simulink model "sergio_arm"  (Simulink 8.5)
settings: Solver=ode45  StartTime=0.0  StopTime=10.0  RelTol=1e-3
undefined symbols (not defined in the file): CPT_w1, GR_w1
libraries: SOEM_EtherCAT_Lib x3
settings Model: Creator=baetenmjj  LastModifiedBy=baetenmjj
settings DataIOCC: SignalLoggingSaveFormat=Dataset
settings OptimizationCC: ExpressionDepthLimit=128
settings DebuggingCC: UnderspecifiedInitializationDetection=Simplified  MergeDetectMultiDrivingBlocksExec=error  FcnCallInpInsideContextMsg=EnableAllAsError  StateNameClashWarn=none
settings GRTTargetCC: CombineOutputUpdateFcns=on  GRTInterface=off

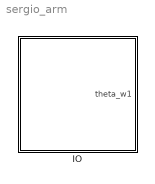
== system sergio_arm ==
  IO : Subsystem

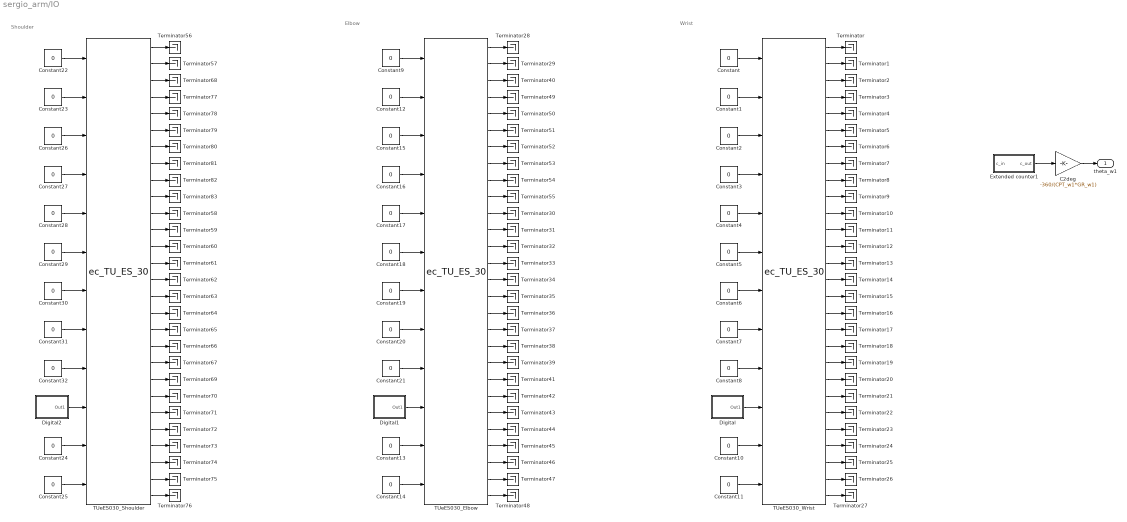
== system sergio_arm/IO ==
  note: Shoulder
  note: Wrist
  note: Elbow
  C2deg : Gain  Gain=-360/(CPT_w1*GR_w1)
  Constant{,1..32} (33 alike) : Constant  Value=0
  Digital : Subsystem
  Digital1 : Subsystem
  Digital2 : Subsystem
  Extended counter1 : Subsystem
  TUeES030_Elbow : SOEM_EtherCAT_Lib/ec_TU_ES_30  link_id=2  slave_num=3  resistance=[1.511, 1.53+0.45*2, 1.53+0.45*2]  kv=[0.0259, 0.0208, 0.0208]  pgain=[4.00, 4.00, 4.00]  igain=[50.00, 50.00, 50.00]  ilimit=[1.0, 1.0, 1.0]  encdir=[1, 1, 1]  encres=[2000, 500, 500]  czero=[17330, 8633, 8522]
  TUeES030_Shoulder : SOEM_EtherCAT_Lib/ec_TU_ES_30  link_id=1  slave_num=2  resistance=[0.611+0.45*2, 1.0, 0.611+0.45*2]  kv=[0.0259, 0, 0.0259]  pgain=[4.00, 0.00, 4.00]  igain=[50.00, 0.00, 50.00]  ilimit=[1.0, 1.0, 1.0]  encdir=[1, 1, 1]  encres=[2000, 2000, 2000]  czero=[17230, 8633, 8526]
  TUeES030_Wrist : SOEM_EtherCAT_Lib/ec_TU_ES_30  link_id=3  slave_num=4  resistance=[0.0, 0, 0]  kv=[0.0, 0, 0]  pgain=[0.00, 10.00, 0.00]  igain=[0.00, 5.00, 0.00]  ilimit=[1.0, 1.0, 1.0]  encdir=[1, 1, -1]  encres=[1024, 512, 512]  czero=[17230, 8835, 8775]
  Terminator{,1..83} (84 alike) : Terminator
  theta_w1 : Outport
  wires:
  Constant27/1 -> TUeES030_Shoulder/4
  Constant29/1 -> TUeES030_Shoulder/6
  Constant30/1 -> TUeES030_Shoulder/7
  TUeES030_Wrist/16 -> Terminator15/1
  Digital2/1(Out1) -> TUeES030_Shoulder/10
  Constant31/1 -> TUeES030_Shoulder/8
  TUeES030_Shoulder/11 -> Terminator58/1
  Constant7/1 -> TUeES030_Wrist/8
  Constant11/1 -> TUeES030_Wrist/12
  Constant6/1 -> TUeES030_Wrist/7
  TUeES030_Shoulder/24 -> Terminator72/1
  TUeES030_Wrist/8 -> Terminator7/1
  TUeES030_Wrist/4 -> Terminator3/1
  TUeES030_Shoulder/1 -> Terminator56/1
  Constant5/1 -> TUeES030_Wrist/6
  Constant25/1 -> TUeES030_Shoulder/12
  TUeES030_Shoulder/2 -> Terminator57/1
  TUeES030_Shoulder/9 -> Terminator82/1
  TUeES030_Wrist/5 -> Terminator4/1
  TUeES030_Shoulder/7 -> Terminator80/1
  TUeES030_Shoulder/8 -> Terminator81/1
  TUeES030_Shoulder/13 -> Terminator60/1
  TUeES030_Wrist/1 -> Terminator/1
  TUeES030_Wrist/11 -> Terminator10/1
  TUeES030_Wrist/17 -> Terminator16/1
  Constant3/1 -> TUeES030_Wrist/4
  TUeES030_Shoulder/18 -> Terminator65/1
  TUeES030_Wrist/7 -> Terminator6/1
  TUeES030_Shoulder/12 -> Terminator59/1
  TUeES030_Shoulder/15 -> Terminator62/1
  TUeES030_Shoulder/6 -> Terminator79/1
  TUeES030_Shoulder/4 -> Terminator77/1
  TUeES030_Shoulder/27 -> Terminator75/1
  TUeES030_Shoulder/22 -> Terminator70/1
  TUeES030_Wrist/12 -> Terminator11/1
  TUeES030_Wrist/14 -> Terminator13/1
  TUeES030_Shoulder/21 -> Terminator69/1
  TUeES030_Shoulder/28 -> Terminator76/1
  Constant24/1 -> TUeES030_Shoulder/11
  TUeES030_Wrist/9 -> Terminator8/1
  Constant32/1 -> TUeES030_Shoulder/9
  TUeES030_Shoulder/20 -> Terminator67/1
  Constant8/1 -> TUeES030_Wrist/9
  Constant/1 -> TUeES030_Wrist/1
  TUeES030_Shoulder/19 -> Terminator66/1
  TUeES030_Wrist/13 -> Terminator12/1
  Constant10/1 -> TUeES030_Wrist/11
  TUeES030_Shoulder/14 -> Terminator61/1
  TUeES030_Shoulder/3 -> Terminator68/1
  TUeES030_Shoulder/10 -> Terminator83/1
  TUeES030_Wrist/3 -> Terminator2/1
  TUeES030_Shoulder/25 -> Terminator73/1
  TUeES030_Wrist/6 -> Terminator5/1
  TUeES030_Shoulder/26 -> Terminator74/1
  Constant2/1 -> TUeES030_Wrist/3
  TUeES030_Wrist/2 -> Terminator1/1
  TUeES030_Shoulder/5 -> Terminator78/1
  TUeES030_Wrist/15 -> Terminator14/1
  Constant1/1 -> TUeES030_Wrist/2
  Constant4/1 -> TUeES030_Wrist/5
  TUeES030_Shoulder/16 -> Terminator63/1
  TUeES030_Wrist/10 -> Terminator9/1
  TUeES030_Shoulder/17 -> Terminator64/1
  TUeES030_Shoulder/23 -> Terminator71/1
  Constant28/1 -> TUeES030_Shoulder/5
  Constant23/1 -> TUeES030_Shoulder/2
  Constant26/1 -> TUeES030_Shoulder/3
  Constant22/1 -> TUeES030_Shoulder/1
  TUeES030_Elbow/26 -> Terminator46/1
  TUeES030_Elbow/24 -> Terminator44/1
  TUeES030_Elbow/27 -> Terminator47/1
  TUeES030_Elbow/25 -> Terminator45/1
  TUeES030_Elbow/28 -> Terminator48/1
  TUeES030_Elbow/23 -> Terminator43/1
  TUeES030_Elbow/17 -> Terminator36/1
  TUeES030_Elbow/18 -> Terminator37/1
  TUeES030_Elbow/22 -> Terminator42/1
  TUeES030_Elbow/21 -> Terminator41/1
  TUeES030_Elbow/19 -> Terminator38/1
  TUeES030_Elbow/20 -> Terminator39/1
  TUeES030_Elbow/3 -> Terminator40/1
  TUeES030_Elbow/13 -> Terminator32/1
  TUeES030_Elbow/16 -> Terminator35/1
  TUeES030_Elbow/12 -> Terminator31/1
  TUeES030_Elbow/8 -> Terminator53/1
  TUeES030_Elbow/5 -> Terminator50/1
  TUeES030_Elbow/4 -> Terminator49/1
  TUeES030_Elbow/11 -> Terminator30/1
  TUeES030_Elbow/15 -> Terminator34/1
  TUeES030_Elbow/1 -> Terminator28/1
  TUeES030_Elbow/14 -> Terminator33/1
  Constant9/1 -> TUeES030_Elbow/1
  TUeES030_Elbow/9 -> Terminator54/1
  TUeES030_Elbow/2 -> Terminator29/1
  TUeES030_Elbow/10 -> Terminator55/1
  TUeES030_Elbow/6 -> Terminator51/1
  TUeES030_Elbow/7 -> Terminator52/1
  TUeES030_Wrist/18 -> Terminator17/1
  TUeES030_Wrist/19 -> Terminator18/1
  TUeES030_Wrist/24 -> Terminator23/1
  TUeES030_Wrist/27 -> Terminator26/1
  TUeES030_Wrist/28 -> Terminator27/1
  TUeES030_Wrist/23 -> Terminator22/1
  TUeES030_Wrist/20 -> Terminator19/1
  TUeES030_Wrist/21 -> Terminator20/1
  TUeES030_Wrist/22 -> Terminator21/1
  TUeES030_Wrist/25 -> Terminator24/1
  TUeES030_Wrist/26 -> Terminator25/1
  Digital/1(Out1) -> TUeES030_Wrist/10
  Constant20/1 -> TUeES030_Elbow/8
  Constant14/1 -> TUeES030_Elbow/12
  Constant19/1 -> TUeES030_Elbow/7
  Constant18/1 -> TUeES030_Elbow/6
  Constant16/1 -> TUeES030_Elbow/4
  Constant21/1 -> TUeES030_Elbow/9
  Constant13/1 -> TUeES030_Elbow/11
  Constant15/1 -> TUeES030_Elbow/3
  Constant12/1 -> TUeES030_Elbow/2
  Constant17/1 -> TUeES030_Elbow/5
  Digital1/1(Out1) -> TUeES030_Elbow/10
  Extended counter1/1(c_out) -> C2deg/1
  C2deg/1 -> theta_w1/1

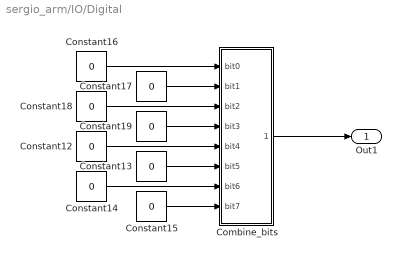
== system sergio_arm/IO/Digital ==
  Combine_bits : Subsystem
  Constant{12..19} (8 alike) : Constant  Value=0
  Out1 : Outport
  wires:
  Constant16/1 -> Combine_bits/1(bit0)
  Constant17/1 -> Combine_bits/2(bit1)
  Constant18/1 -> Combine_bits/3(bit2)
  Constant19/1 -> Combine_bits/4(bit3)
  Constant12/1 -> Combine_bits/5(bit4)
  Constant13/1 -> Combine_bits/6(bit5)
  Constant14/1 -> Combine_bits/7(bit6)
  Constant15/1 -> Combine_bits/8(bit7)
  Combine_bits/1(Out1) -> Out1/1

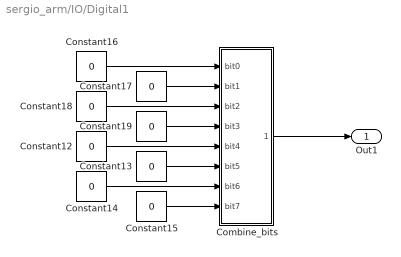
== system sergio_arm/IO/Digital1 ==
  Combine_bits : Subsystem
  Constant{12..19} (8 alike) : Constant  Value=0
  Out1 : Outport
  wires:
  Constant16/1 -> Combine_bits/1(bit0)
  Constant17/1 -> Combine_bits/2(bit1)
  Constant18/1 -> Combine_bits/3(bit2)
  Constant19/1 -> Combine_bits/4(bit3)
  Constant12/1 -> Combine_bits/5(bit4)
  Constant13/1 -> Combine_bits/6(bit5)
  Constant14/1 -> Combine_bits/7(bit6)
  Constant15/1 -> Combine_bits/8(bit7)
  Combine_bits/1(Out1) -> Out1/1

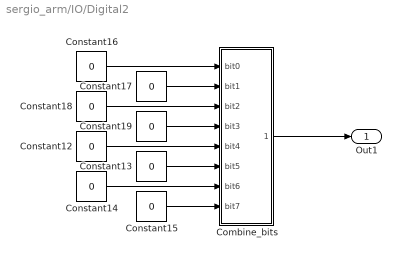
== system sergio_arm/IO/Digital2 ==
  Combine_bits : Subsystem
  Constant{12..19} (8 alike) : Constant  Value=0
  Out1 : Outport
  wires:
  Constant16/1 -> Combine_bits/1(bit0)
  Constant17/1 -> Combine_bits/2(bit1)
  Constant18/1 -> Combine_bits/3(bit2)
  Constant19/1 -> Combine_bits/4(bit3)
  Constant12/1 -> Combine_bits/5(bit4)
  Constant13/1 -> Combine_bits/6(bit5)
  Constant14/1 -> Combine_bits/7(bit6)
  Constant15/1 -> Combine_bits/8(bit7)
  Combine_bits/1(Out1) -> Out1/1

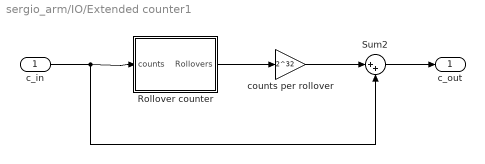
== system sergio_arm/IO/Extended counter1 ==
  c_in : Inport
  Rollover counter : Subsystem
  Sum2 : Sum  Inputs=|++
  counts per rollover : Gain  Gain=2^32
  c_out : Outport
  wires:
  counts per rollover/1 -> Sum2/1
  Rollover counter/1(Rollovers) -> counts per rollover/1
  c_in/1 -> Rollover counter/1(counts), Sum2/2
  Sum2/1 -> c_out/1

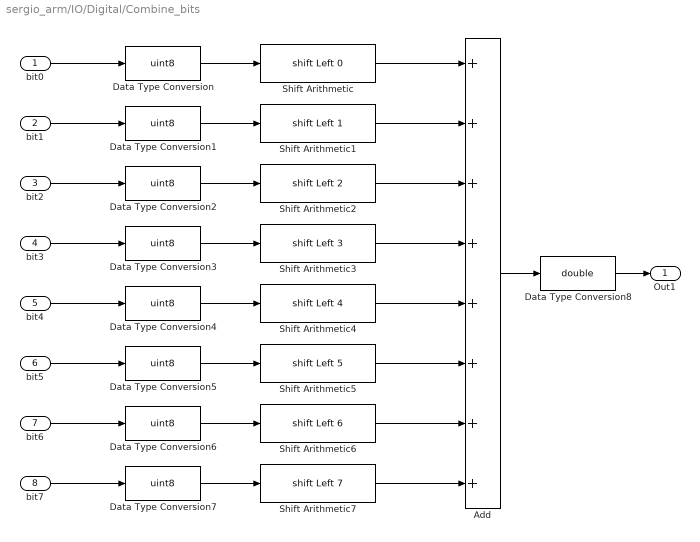
== system sergio_arm/IO/Digital/Combine_bits ==
  bit0 : Inport
  bit1 : Inport  Port=2
  bit2 : Inport  Port=3
  bit3 : Inport  Port=4
  bit4 : Inport  Port=5
  bit5 : Inport  Port=6
  bit6 : Inport  Port=7
  bit7 : Inport  Port=8
  Add : Sum  Inputs=++++++++
  Data Type Conversion{,1..7} (8 alike) : DataTypeConversion  OutDataTypeStr=uint8
  Data Type Conversion8 : DataTypeConversion  OutDataTypeStr=double
  Shift Arithmetic : ArithShift  BitShiftDirection=Left
  Shift Arithmetic1 : ArithShift  BitShiftNumber=1  BitShiftDirection=Left
  Shift Arithmetic2 : ArithShift  BitShiftNumber=2  BitShiftDirection=Left
  Shift Arithmetic3 : ArithShift  BitShiftNumber=3  BitShiftDirection=Left
  Shift Arithmetic4 : ArithShift  BitShiftNumber=4  BitShiftDirection=Left
  Shift Arithmetic5 : ArithShift  BitShiftNumber=5  BitShiftDirection=Left
  Shift Arithmetic6 : ArithShift  BitShiftNumber=6  BitShiftDirection=Left
  Shift Arithmetic7 : ArithShift  BitShiftNumber=7  BitShiftDirection=Left
  Out1 : Outport
  wires:
  bit0/1 -> Data Type Conversion/1
  bit1/1 -> Data Type Conversion1/1
  bit2/1 -> Data Type Conversion2/1
  bit3/1 -> Data Type Conversion3/1
  bit4/1 -> Data Type Conversion4/1
  bit5/1 -> Data Type Conversion5/1
  bit6/1 -> Data Type Conversion6/1
  bit7/1 -> Data Type Conversion7/1
  Data Type Conversion/1 -> Shift Arithmetic/1
  Data Type Conversion1/1 -> Shift Arithmetic1/1
  Data Type Conversion2/1 -> Shift Arithmetic2/1
  Data Type Conversion3/1 -> Shift Arithmetic3/1
  Data Type Conversion4/1 -> Shift Arithmetic4/1
  Data Type Conversion5/1 -> Shift Arithmetic5/1
  Data Type Conversion6/1 -> Shift Arithmetic6/1
  Data Type Conversion7/1 -> Shift Arithmetic7/1
  Shift Arithmetic/1 -> Add/1
  Shift Arithmetic1/1 -> Add/2
  Shift Arithmetic2/1 -> Add/3
  Shift Arithmetic3/1 -> Add/4
  Shift Arithmetic4/1 -> Add/5
  Shift Arithmetic5/1 -> Add/6
  Shift Arithmetic6/1 -> Add/7
  Shift Arithmetic7/1 -> Add/8
  Add/1 -> Data Type Conversion8/1
  Data Type Conversion8/1 -> Out1/1

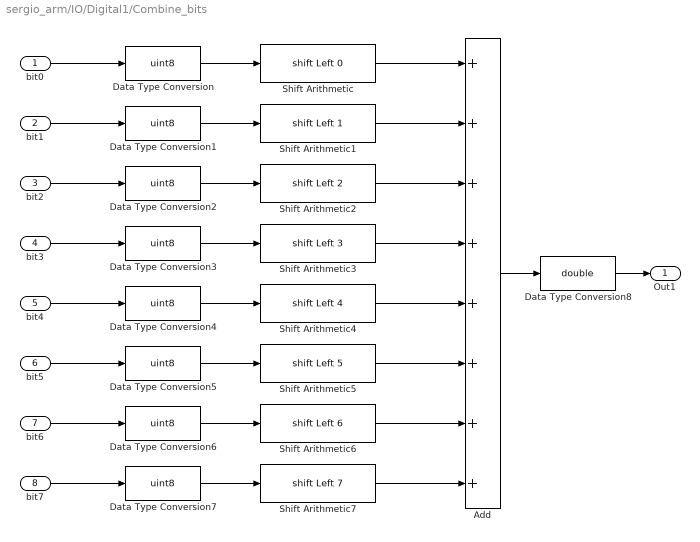
== system sergio_arm/IO/Digital1/Combine_bits ==
  bit0 : Inport
  bit1 : Inport  Port=2
  bit2 : Inport  Port=3
  bit3 : Inport  Port=4
  bit4 : Inport  Port=5
  bit5 : Inport  Port=6
  bit6 : Inport  Port=7
  bit7 : Inport  Port=8
  Add : Sum  Inputs=++++++++
  Data Type Conversion{,1..7} (8 alike) : DataTypeConversion  OutDataTypeStr=uint8
  Data Type Conversion8 : DataTypeConversion  OutDataTypeStr=double
  Shift Arithmetic : ArithShift  BitShiftDirection=Left
  Shift Arithmetic1 : ArithShift  BitShiftNumber=1  BitShiftDirection=Left
  Shift Arithmetic2 : ArithShift  BitShiftNumber=2  BitShiftDirection=Left
  Shift Arithmetic3 : ArithShift  BitShiftNumber=3  BitShiftDirection=Left
  Shift Arithmetic4 : ArithShift  BitShiftNumber=4  BitShiftDirection=Left
  Shift Arithmetic5 : ArithShift  BitShiftNumber=5  BitShiftDirection=Left
  Shift Arithmetic6 : ArithShift  BitShiftNumber=6  BitShiftDirection=Left
  Shift Arithmetic7 : ArithShift  BitShiftNumber=7  BitShiftDirection=Left
  Out1 : Outport
  wires:
  bit0/1 -> Data Type Conversion/1
  bit1/1 -> Data Type Conversion1/1
  bit2/1 -> Data Type Conversion2/1
  bit3/1 -> Data Type Conversion3/1
  bit4/1 -> Data Type Conversion4/1
  bit5/1 -> Data Type Conversion5/1
  bit6/1 -> Data Type Conversion6/1
  bit7/1 -> Data Type Conversion7/1
  Data Type Conversion/1 -> Shift Arithmetic/1
  Data Type Conversion1/1 -> Shift Arithmetic1/1
  Data Type Conversion2/1 -> Shift Arithmetic2/1
  Data Type Conversion3/1 -> Shift Arithmetic3/1
  Data Type Conversion4/1 -> Shift Arithmetic4/1
  Data Type Conversion5/1 -> Shift Arithmetic5/1
  Data Type Conversion6/1 -> Shift Arithmetic6/1
  Data Type Conversion7/1 -> Shift Arithmetic7/1
  Shift Arithmetic/1 -> Add/1
  Shift Arithmetic1/1 -> Add/2
  Shift Arithmetic2/1 -> Add/3
  Shift Arithmetic3/1 -> Add/4
  Shift Arithmetic4/1 -> Add/5
  Shift Arithmetic5/1 -> Add/6
  Shift Arithmetic6/1 -> Add/7
  Shift Arithmetic7/1 -> Add/8
  Add/1 -> Data Type Conversion8/1
  Data Type Conversion8/1 -> Out1/1

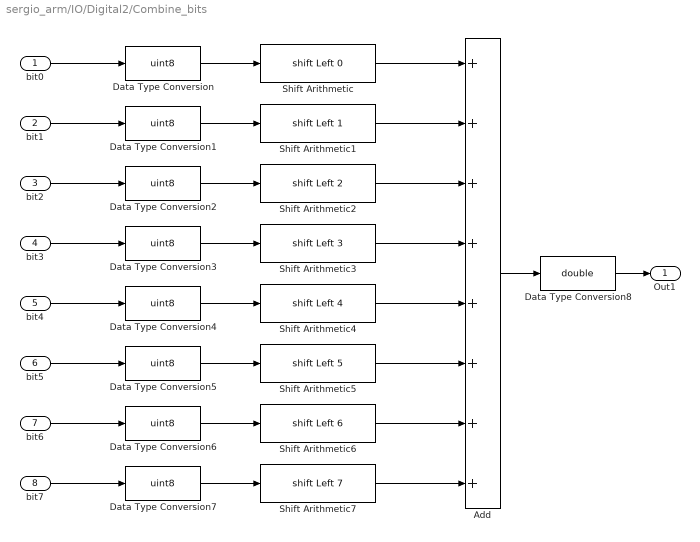
== system sergio_arm/IO/Digital2/Combine_bits ==
  bit0 : Inport
  bit1 : Inport  Port=2
  bit2 : Inport  Port=3
  bit3 : Inport  Port=4
  bit4 : Inport  Port=5
  bit5 : Inport  Port=6
  bit6 : Inport  Port=7
  bit7 : Inport  Port=8
  Add : Sum  Inputs=++++++++
  Data Type Conversion{,1..7} (8 alike) : DataTypeConversion  OutDataTypeStr=uint8
  Data Type Conversion8 : DataTypeConversion  OutDataTypeStr=double
  Shift Arithmetic : ArithShift  BitShiftDirection=Left
  Shift Arithmetic1 : ArithShift  BitShiftNumber=1  BitShiftDirection=Left
  Shift Arithmetic2 : ArithShift  BitShiftNumber=2  BitShiftDirection=Left
  Shift Arithmetic3 : ArithShift  BitShiftNumber=3  BitShiftDirection=Left
  Shift Arithmetic4 : ArithShift  BitShiftNumber=4  BitShiftDirection=Left
  Shift Arithmetic5 : ArithShift  BitShiftNumber=5  BitShiftDirection=Left
  Shift Arithmetic6 : ArithShift  BitShiftNumber=6  BitShiftDirection=Left
  Shift Arithmetic7 : ArithShift  BitShiftNumber=7  BitShiftDirection=Left
  Out1 : Outport
  wires:
  bit0/1 -> Data Type Conversion/1
  bit1/1 -> Data Type Conversion1/1
  bit2/1 -> Data Type Conversion2/1
  bit3/1 -> Data Type Conversion3/1
  bit4/1 -> Data Type Conversion4/1
  bit5/1 -> Data Type Conversion5/1
  bit6/1 -> Data Type Conversion6/1
  bit7/1 -> Data Type Conversion7/1
  Data Type Conversion/1 -> Shift Arithmetic/1
  Data Type Conversion1/1 -> Shift Arithmetic1/1
  Data Type Conversion2/1 -> Shift Arithmetic2/1
  Data Type Conversion3/1 -> Shift Arithmetic3/1
  Data Type Conversion4/1 -> Shift Arithmetic4/1
  Data Type Conversion5/1 -> Shift Arithmetic5/1
  Data Type Conversion6/1 -> Shift Arithmetic6/1
  Data Type Conversion7/1 -> Shift Arithmetic7/1
  Shift Arithmetic/1 -> Add/1
  Shift Arithmetic1/1 -> Add/2
  Shift Arithmetic2/1 -> Add/3
  Shift Arithmetic3/1 -> Add/4
  Shift Arithmetic4/1 -> Add/5
  Shift Arithmetic5/1 -> Add/6
  Shift Arithmetic6/1 -> Add/7
  Shift Arithmetic7/1 -> Add/8
  Add/1 -> Data Type Conversion8/1
  Data Type Conversion8/1 -> Out1/1

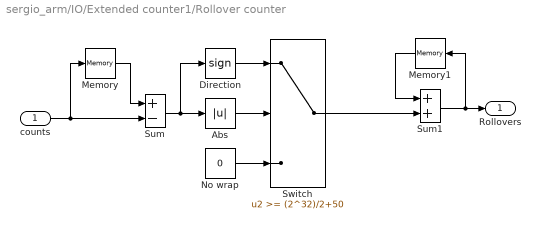
== system sergio_arm/IO/Extended counter1/Rollover counter ==
  counts : Inport
  Abs : Abs
  Direction : Signum
  Memory : Memory  X0=2^32/2  InheritSampleTime=on
  Memory1 : Memory
  No wrap : Constant  Value=0
  Sum : Sum  Inputs=+-
  Sum1 : Sum
  Switch : Switch  Threshold=(2^32)/2+50
  Rollovers : Outport
  wires:
  Memory1/1 -> Sum1/1
  Sum1/1 -> Memory1/1, Rollovers/1
  Switch/1 -> Sum1/2
  Direction/1 -> Switch/1
  No wrap/1 -> Switch/3
  Abs/1 -> Switch/2
  Sum/1 -> Abs/1, Direction/1
  Memory/1 -> Sum/1
  counts/1 -> Sum/2, Memory/1
